simulink model "simpleObserver"  (R2021b)
settings: Solver=ode1  StartTime=0.0  StopTime=Inf  FixedStep=0.01  RelTol=1e-3
libraries: TcTargetLib x12
settings Model: SimulationMode=external  Creator=ATLabor  LastModifiedBy=ATLabor
settings OptimizationCC: LocalBlockOutputs=off
settings RTWCC: Description=TwinCAT GRT Target  SystemTargetFile=TwinCatGrt.tlc  GenCodeOnly=on  TemplateMakefile=tcgrt_msbuild.tmf  TargetLang=C++
settings STFCustomTargetCC: TargetLangStandard=C++11 (ISO)  CombineOutputUpdateFcns=on  CPPClassGenCompliant=on  GRTInterface=off  SystemTargetFile=TwinCatGrt.tlc
settings GRTTargetCC: TargetLangStandard=C++11 (ISO)  ParMdlRefBuildCompliant=off  CompOptLevelCompliant=off  ConcurrentExecutionCompliant=off  MatFileLogging=off  UseToolchainInfoCompliant=off  ExtModeMexFile=TcExtModeClient

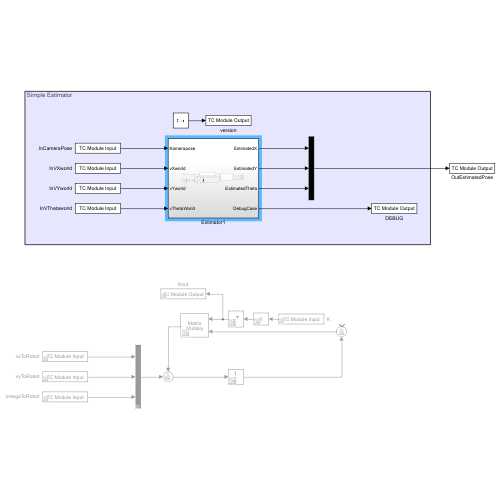
[thumbnail: Simulink's stored preview of the top-level diagram]
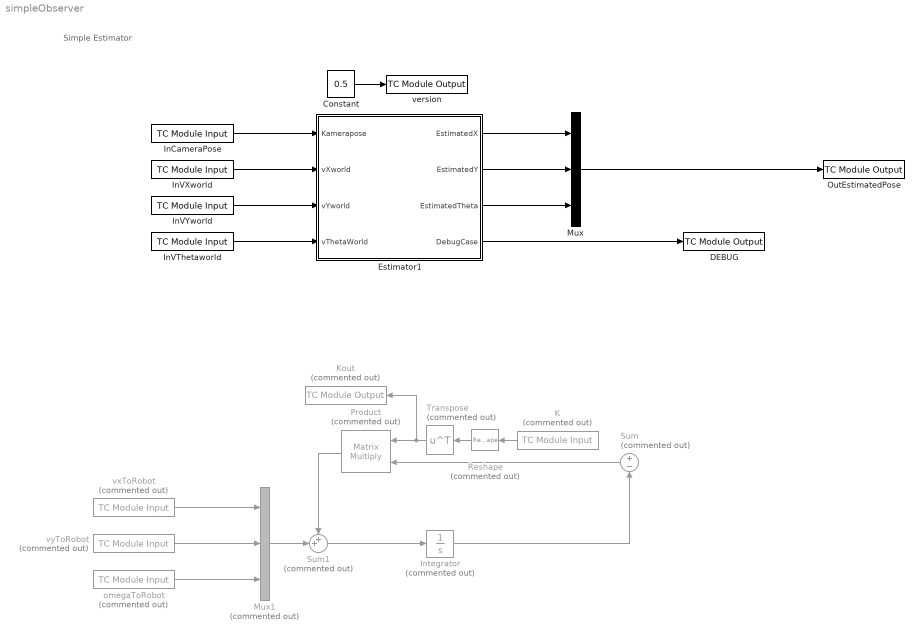
== system simpleObserver ==
  note: Simple Estimator
  Constant : Constant  Value=0.5
  DEBUG : TcTargetLib/TC Module Output  PortDataType=double  PortDim=1  SampleTime=-1  CodeGenConnectType=DataArea (OutputSrc)  DataTypeOverride=off
      settings: SourceProductName=Beckhoff TwinCAT Target
  Estimator1 : Subsystem
  InCameraPose : TcTargetLib/TC Module Input  PortDataType=double  PortDim=3  Value=[0 0 0]  SampleTime=-1  CodeGenConnectType=DataArea (InputDst)  DataTypeOverride=on
      settings: SourceProductName=Beckhoff TwinCAT Target
  InVThetaworld : TcTargetLib/TC Module Input  PortDataType=double  PortDim=1  Value=0  SampleTime=-1  CodeGenConnectType=DataArea (InputDst)  DataTypeOverride=off
      settings: SourceProductName=Beckhoff TwinCAT Target
  InVXworld : TcTargetLib/TC Module Input  PortDataType=double  PortDim=1  Value=0  SampleTime=-1  CodeGenConnectType=DataArea (InputDst)  DataTypeOverride=off
      settings: SourceProductName=Beckhoff TwinCAT Target
  InVYworld : TcTargetLib/TC Module Input  PortDataType=double  PortDim=1  Value=0  SampleTime=-1  CodeGenConnectType=DataArea (InputDst)  DataTypeOverride=off
      settings: SourceProductName=Beckhoff TwinCAT Target
  Integrator : Integrator  Commented=on
  K : TcTargetLib/TC Module Input  Commented=on  PortDataType=double  PortDim=[3,3]  Value=[1,0,0;0,1,0;0,0,1]  SampleTime=-1  CodeGenConnectType=DataArea (InputDst)  DataTypeOverride=off
      settings: SourceProductName=Beckhoff TwinCAT Target
  Kout : TcTargetLib/TC Module Output  Commented=on  PortDataType=double  PortDim=[3,3]  SampleTime=-1  CodeGenConnectType=DataArea (OutputSrc)  DataTypeOverride=off
      settings: SourceProductName=Beckhoff TwinCAT Target
  Mux : Mux  Inputs=3
  Mux1 : Mux  Commented=on  Inputs=3
  OutEstimatedPose : TcTargetLib/TC Module Output  PortDataType=double  PortDim=3  SampleTime=-1  CodeGenConnectType=DataArea (OutputSrc)  DataTypeOverride=off
      settings: SourceProductName=Beckhoff TwinCAT Target
  Product : Product  Commented=on  Multiplication=Matrix(*)
  Reshape : Reshape  Commented=on  OutputDimensionality=Customize  OutputDimensions=[3,3]
  Sum : Sum  Commented=on  Inputs=+|-
  Sum1 : Sum  Commented=on  Inputs=++|
  Transpose : Math  Commented=on  Operator=transpose  SaturateOnIntegerOverflow=on
  omegaToRobot : TcTargetLib/TC Module Input  Commented=on  PortDataType=double  PortDim=1  Value=0  SampleTime=-1  CodeGenConnectType=DataArea (InputDst)  DataTypeOverride=off
      settings: SourceProductName=Beckhoff TwinCAT Target
  version : TcTargetLib/TC Module Output  PortDataType=double  PortDim=1  SampleTime=-1  CodeGenConnectType=DataArea (OutputSrc)  DataTypeOverride=off
      settings: SourceProductName=Beckhoff TwinCAT Target
  vxToRobot : TcTargetLib/TC Module Input  Commented=on  PortDataType=double  PortDim=1  Value=0  SampleTime=-1  CodeGenConnectType=DataArea (InputDst)  DataTypeOverride=off
      settings: SourceProductName=Beckhoff TwinCAT Target
  vyToRobot : TcTargetLib/TC Module Input  Commented=on  PortDataType=double  PortDim=1  Value=0  SampleTime=-1  CodeGenConnectType=DataArea (InputDst)  DataTypeOverride=off
      settings: SourceProductName=Beckhoff TwinCAT Target
  wires:
  Estimator1/3(EstimatedTheta) -> Mux/3
  Constant/1 -> version/1
  InVYworld/1 -> Estimator1/3(vYworld)
  Estimator1/1(EstimatedX) -> Mux/1
  Estimator1/2(EstimatedY) -> Mux/2
  InVXworld/1 -> Estimator1/2(vXworld)
  InVThetaworld/1 -> Estimator1/4(vThetaWorld)
  InCameraPose/1 -> Estimator1/1(Kamerapose)
  Estimator1/4(DebugCase) -> DEBUG/1
  Integrator/1 -> Sum/2
  vxToRobot/1 -> Mux1/1
  omegaToRobot/1 -> Mux1/3
  vyToRobot/1 -> Mux1/2
  Sum1/1 -> Integrator/1
  Mux1/1 -> Sum1/2
  Sum/1 -> Product/2
  Product/1 -> Sum1/1
  K/1 -> Reshape/1
  Reshape/1 -> Transpose/1
  Transpose/1 -> Kout/1, Product/1
  Mux/1 -> OutEstimatedPose/1

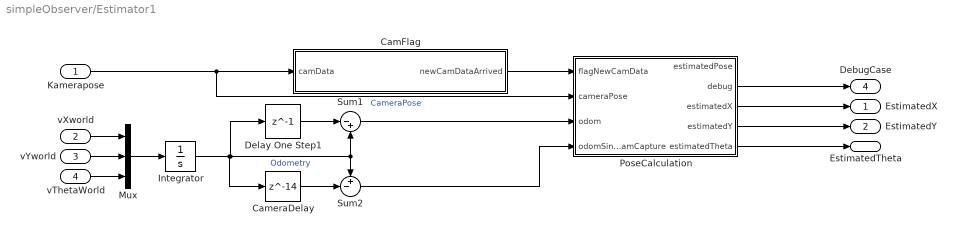
== system simpleObserver/Estimator1 ==
  Kamerapose : Inport
  vXworld : Inport  Port=2
  vYworld : Inport  Port=3
  vThetaWorld : Inport  Port=4
  CamFlag : MATLAB Function  TreatAsAtomicUnit=on
  CameraDelay : Delay  DelayLength=14
  Delay One Step1 : Delay  DelayLength=1
  Integrator : Integrator
  Mux : Mux  Inputs=3
  PoseCalculation : MATLAB Function  TreatAsAtomicUnit=on
  Sum1 : Sum  Inputs=|-+
  Sum2 : Sum  Inputs=+-|
  EstimatedX : Outport
  EstimatedY : Outport  Port=2
  EstimatedTheta : Outport  Port=3
  DebugCase : Outport  Port=4
  wires:
  vThetaWorld/1 -> Mux/3
  Sum2/1 -> PoseCalculation/4(odomSinceCamCapture)
  vXworld/1 -> Mux/1
  Kamerapose/1 -> PoseCalculation/2(cameraPose), CamFlag/1(camData)  "CameraPose"
  Integrator/1 -> Sum1/2, Sum2/1, Delay One Step1/1, CameraDelay/1  "Odometry"
  vYworld/1 -> Mux/2
  CamFlag/1(newCamDataArrived) -> PoseCalculation/1(flagNewCamData)
  Delay One Step1/1 -> Sum1/1
  Sum1/1 -> PoseCalculation/3(odom)
  PoseCalculation/2(debug) -> DebugCase/1
  PoseCalculation/4(estimatedY) -> EstimatedY/1
  PoseCalculation/3(estimatedX) -> EstimatedX/1
  PoseCalculation/5(estimatedTheta) -> EstimatedTheta/1
  Mux/1 -> Integrator/1
  CameraDelay/1 -> Sum2/2

== matlab function simpleObserver/Estimator1/CamFlag ==
  data: camData input; newCamDataArrived output
function newCamDataArrived = fcn(camData)

persistent oldCamData

if isempty(oldCamData)
    oldCamData = [0 0 0]';
end

if any(camData(1:2)) && camData ~= oldCamData
    newCamDataArrived = true;
else
    newCamDataArrived = false;
    oldCamData = camData;
end

== matlab function simpleObserver/Estimator1/PoseCalculation ==
  settings: updateMethod=DISCRETE
  data: flagNewCamData input; cameraPose input; estimatedPose output; odom input; odomSinceCamCapture input; debug output; estimatedX output; estimatedY output; estimatedTheta output
function [estimatedPose, debug, estimatedX, estimatedY, estimatedTheta]= fcn(flagNewCamData, cameraPose, odom, odomSinceCamCapture)

% Variables
persistent estPoseOld

if isempty(estPoseOld)
    estPoseOld = [0 0 0]';
end

% Case 1: Camera Flag is set (New Cameradata) and CameraData is valid
if flagNewCamData == 1
    estimatedPose = cameraPose(1:3) + odomSinceCamCapture;   %OdomSinceCamCapture describes the pose changes since the camera captured the position because the camera data is delayed. in this time the robot drives further.
    estPoseOld = estimatedPose;
    debug = 1;

    % Case 2: No new Cameradata or invalid Cmeradata (integrate transformed velocities of
    % roboter in worldframe
else
    estimatedPose = estPoseOld + odom;
    estPoseOld = estimatedPose;  
    debug =2;
end

estimatedX = estimatedPose(1);
estimatedY = estimatedPose(2);
estimatedTheta = estimatedPose(3);
